simulink model "RLC_circuit"  (R2015a)
settings: Solver=ode45  StartTime=0.0  StopTime=10  RelTol=1e-3
undefined symbols (not defined in the file or in its folder): x1, x2
settings Model: Creator=John  LastModifiedBy=John

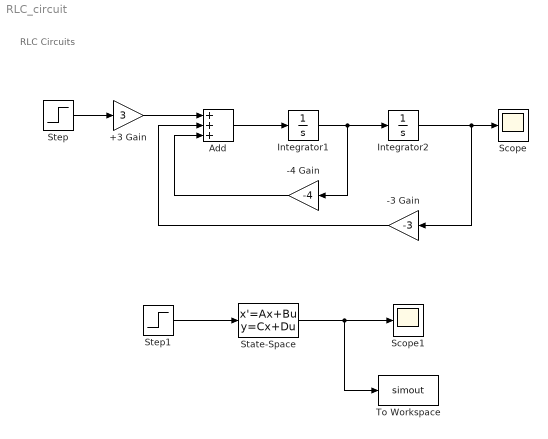
== system RLC_circuit ==
  note: RLC Circuits
  +3 Gain : Gain  Gain=3
  -3 Gain : Gain  Gain=-3
  -4 Gain : Gain  Gain=-4
  Add : Sum  Inputs=+++
  Integrator1 : Integrator
  Integrator2 : Integrator  InitialCondition=0.5
  Scope : Scope
  Scope1 : Scope
  State-Space : StateSpace  A=[4 -4; 3/4 0]  B=[4 0]'  C=[0 1]  D=0  X0=[x1 x2]'
  Step : Step  SampleTime=0
  Step1 : Step  SampleTime=0
  To Workspace : ToWorkspace  VariableName=simout  SaveFormat=Timeseries  SampleTime=-1
  wires:
  +3 Gain/1 -> Add/1
  Add/1 -> Integrator1/1
  Step/1 -> +3 Gain/1
  Integrator1/1 -> -4 Gain/1, Integrator2/1
  Integrator2/1 -> -3 Gain/1, Scope/1
  -3 Gain/1 -> Add/2
  -4 Gain/1 -> Add/3
  Step1/1 -> State-Space/1
  State-Space/1 -> To Workspace/1, Scope1/1
